simulink model "MSD_control"  (R2024b)
settings: Solver=ode4  StartTime=0.0  StopTime=10.0  FixedStep=1e-4  MaxStep=1e-3  RelTol=1e-3  EnableMultiTasking=on
values from neighbouring files (symbols this model uses):
  k_ref = 0.12    [MAIN_MSD_control.m]    (also in MAIN_slip_control.m)
  k_thresh = 0.001    [MAIN_MSD_control.m]    (also in MAIN_slip_control.m)
  Kd_high = 40    [MAIN_MSD_control.m]    (also in MAIN_slip_control.m = 5)
  Kd_low = 30    [MAIN_MSD_control.m]    (also in MAIN_slip_control.m = 5)
  Kd_thresh = 0/3.6    (= 0)    [MAIN_slip_control.m]
  Kp_high = 400    [MAIN_MSD_control.m]    (also in MAIN_slip_control.m = 500)
  Kp_low = 10    [MAIN_MSD_control.m]    (also in MAIN_slip_control.m = 100)
undefined symbols (not defined in the file or in its folder): Kp_thresh, par
libraries: simulink x3, Delft_Tyre_dtlib x1, Delft_Tyre_sm1glib x1
settings Model: Creator=bshyrokau  LastModifiedBy=nicvi
settings SolverCC: AlgebraicLoopSolver=TrustRegion
settings DataIOCC: SaveOutput=off  SignalLogging=off  DSMLogging=off  SaveTime=off  ReturnWorkspaceOutputs=off
settings OptimizationCC: ReuseModelBlockBuffer=off  LifeSpan=inf
settings DebuggingCC: UnconnectedInputMsg=warning  UnconnectedOutputMsg=warning  UnconnectedLineMsg=warning  AllowSymbolicDim=off  SFUnexpectedBacktrackingDiag=warning  SFNoUnconditionalDefaultTransitionDiag=warning  SFExecutionAtInitializationDiag=none  ArithmeticOperatorsInVariantConditions=warning
settings ModelReferenceCC: EnableRefExpFcnMdlSchedulingChecks=on  PropagateSignalLabelsOutOfModel=off
settings SFSimCC: SimUseLocalCustomCode=off  CustomCodeUndefinedFunction=UseInterfaceOnly
settings RTWCC: RTWUseLocalCustomCode=off  GPUComputeCapability=3.5  DLArmComputeVersion=19.05
settings CodeAppCC: StateflowObjectComments=on
settings GRTTargetCC: TargetLangStandard=C89/C90 (ANSI)
settings ConfigComp: CovMetricSettings=dw  CovSaveCumulativeToWorkspaceVar=on  CovSaveSingleToWorkspaceVar=on  CovExternalEMLEnable=off

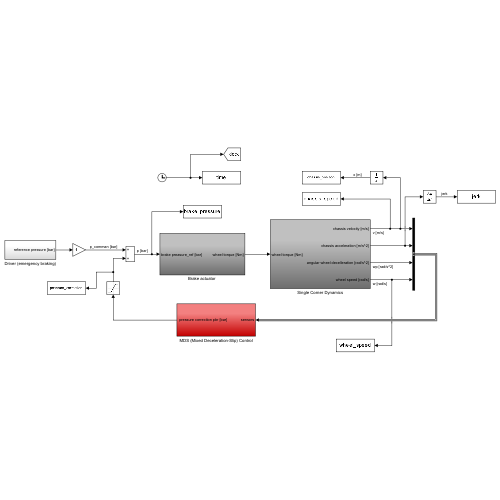
[thumbnail: Simulink's stored preview of the top-level diagram]
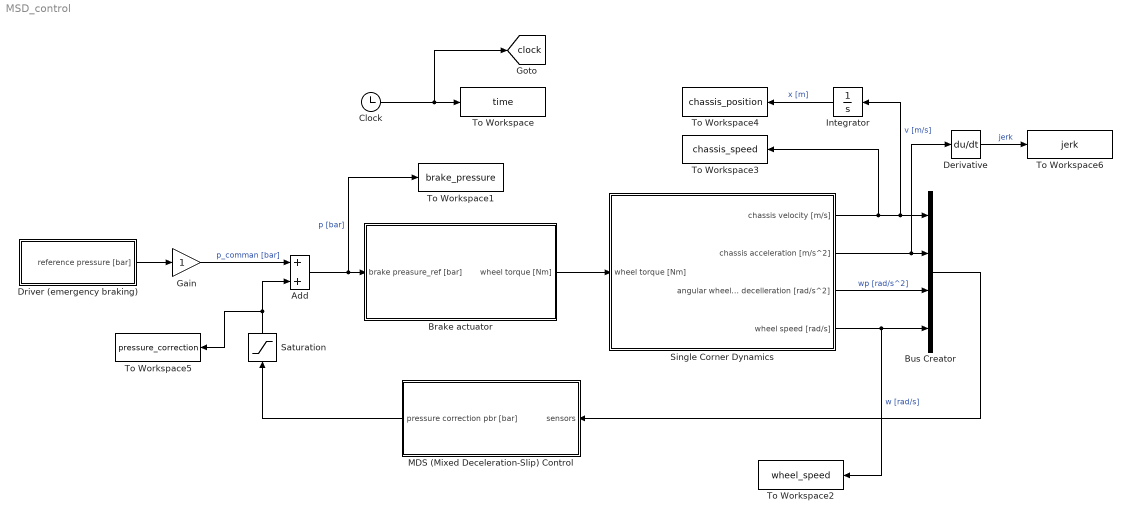
== system MSD_control ==
  Add : Sum
  "Brake actuator " : Subsystem
  Bus Creator : BusCreator  Inputs=4
  Clock : Clock
  Derivative : Derivative
  Driver (emergency braking) : Subsystem
  Gain : Gain
  Integrator : Integrator
  MDS (Mixed Deceleration-Slip) Control : Subsystem
  Saturation : Saturate  UpperLimit=0  LowerLimit=-100
  Single Corner Dynamics : Subsystem
  To Workspace : ToWorkspace  VariableName=time  SampleTime=-1
  To Workspace1 : ToWorkspace  VariableName=brake_pressure  SampleTime=-1
  To Workspace2 : ToWorkspace  VariableName=wheel_speed  SampleTime=-1
  To Workspace3 : ToWorkspace  VariableName=chassis_speed  SampleTime=-1
  To Workspace4 : ToWorkspace  VariableName=chassis_position  SampleTime=-1
  To Workspace5 : ToWorkspace  VariableName=pressure_correction  SampleTime=-1
  To Workspace6 : ToWorkspace  VariableName=jerk  SampleTime=-1
  tag scope: clock=global
  wires:
  "Brake actuator "/1(wheel torque [Nm]) -> Single Corner Dynamics/1(wheel torque [Nm])
  Add/1 -> To Workspace1/1, "Brake actuator "/1(brake preasure_ref [bar])  "p [bar]"
  MDS (Mixed Deceleration-Slip) Control/1(" pressure correction pbr [bar]") -> Saturation/1
  Single Corner Dynamics/1(chassis velocity [m/s]) -> Integrator/1, Bus Creator/1, To Workspace3/1  "v [m/s]"
  Single Corner Dynamics/3(angular wheel decelleration [rad/s^2]) -> Bus Creator/3  "wp [rad/s^2]"
  Single Corner Dynamics/4(wheel speed [rad/s]) -> Bus Creator/4, To Workspace2/1  "w [rad/s]"
  Bus Creator/1 -> MDS (Mixed Deceleration-Slip) Control/1(sensors)
  Driver (emergency braking)/1(reference pressure [bar]) -> Gain/1
  Gain/1 -> Add/1  "p_comman [bar]"
  Clock/1 -> [clock], To Workspace/1
  Saturation/1 -> To Workspace5/1, Add/2
  Integrator/1 -> To Workspace4/1  "x [m]"
  Single Corner Dynamics/2(chassis acceleration [m/s^2]) -> Derivative/1, Bus Creator/2
  Derivative/1 -> To Workspace6/1  "jerk"

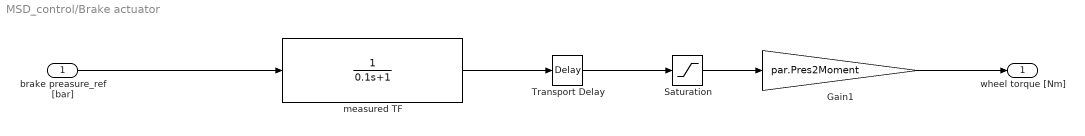
== system MSD_control/Brake actuator  ==
  brake preasure_ref [bar] : Inport
  " measured TF " : TransferFcn  Denominator=[0.1 1]
  Gain1 : Gain  Gain=par.Pres2Moment
  Saturation : Saturate  UpperLimit=par.max_pressure  LowerLimit=0
  Transport Delay : TransportDelay  DelayTime=0.06
  wheel torque [Nm] : Outport  VectorParamsAs1DForOutWhenUnconnected=off
  wires:
  Gain1/1 -> wheel torque [Nm]/1
  " measured TF "/1 -> Transport Delay/1
  Transport Delay/1 -> Saturation/1
  Saturation/1 -> Gain1/1
  brake preasure_ref [bar]/1 -> " measured TF "/1

== system MSD_control/Driver (emergency braking) ==
  Ramp : simulink/Sources/Ramp  slope=100  start=2  InitialOutput=0
  Saturation : Saturate  UpperLimit=100  LowerLimit=0
  reference pressure [bar] : Outport  VectorParamsAs1DForOutWhenUnconnected=off
  wires:
  Ramp/1 -> Saturation/1
  Saturation/1 -> reference pressure [bar]/1

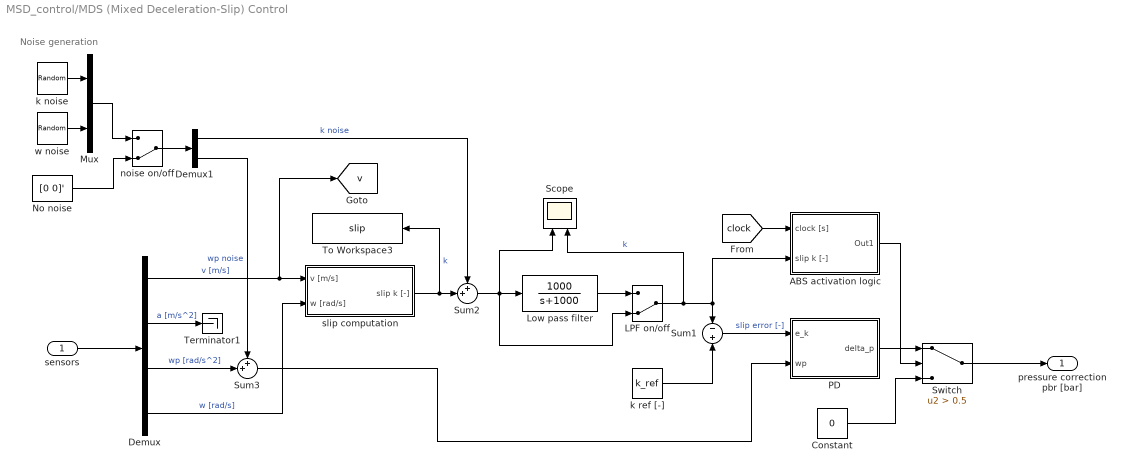
== system MSD_control/MDS (Mixed Deceleration-Slip) Control ==
  note: Noise generation
  sensors : Inport
  ABS activation logic : Subsystem
  Constant : Constant  Value=0
  Demux : Demux
  Demux1 : Demux  Outputs=2
  LPF on/off : ManualSwitch  CurrentSetting=0
  Low pass filter : TransferFcn  Numerator=[1000]  Denominator=[1 1000]
  Mux : Mux  Inputs=2
  No noise : Constant  Value=[0 0]'  OutDataTypeStr=Inherit: Inherit via back propagation
  PD : Subsystem
  Scope : Scope  NumInputPorts=2
  Sum1 : Sum  Inputs=-|+
  Sum2 : Sum  Inputs=++|
  Sum3 : Sum  Inputs=++|
  Switch : Switch  Criteria=u2 > Threshold  Threshold=0.5  SaturateOnIntegerOverflow=off  InputSameDT=off
  Terminator1 : Terminator
  To Workspace3 : ToWorkspace  VariableName=slip  SampleTime=-1
  k noise : UniformRandomNumber  Minimum=-0.025  Maximum=0.025  SampleTime=0
  k ref [-] : Constant  Value=k_ref
  noise on/off : ManualSwitch  CurrentSetting=0
  slip computation : Subsystem
  w noise : UniformRandomNumber  Minimum=-0.5  Maximum=0.5  SampleTime=0
  " pressure correction pbr [bar]" : Outport  VectorParamsAs1DForOutWhenUnconnected=off
  tag scope: v=global
  wires:
  sensors/1 -> Demux/1
  Demux/1 -> [v], slip computation/1(v [m/s])  "v [m/s]"
  Demux/2 -> Terminator1/1  "a [m/s^2]"
  Demux/4 -> slip computation/2(w [rad/s])  "w [rad/s]"
  Demux/3 -> Sum3/2  "wp [rad/s^2]"
  PD/1(delta_p) -> Switch/1
  k ref [-]/1 -> Sum1/2
  Sum1/1 -> PD/1(e_k)  "slip error [-]"
  Switch/1 -> " pressure correction pbr [bar]"/1
  ABS activation logic/1(Out1) -> Switch/2
  Constant/1 -> Switch/3
  [clock] -> ABS activation logic/1(clock [s])
  slip computation/1(slip k [-]) -> To Workspace3/1, Sum2/2  "k"
  w noise/1 -> Mux/2
  Mux/1 -> noise on/off/1
  k noise/1 -> Mux/1
  Demux1/2 -> Sum3/1  "wp noise"
  Demux1/1 -> Sum2/1  "k noise"
  noise on/off/1 -> Demux1/1
  No noise/1 -> noise on/off/2
  Sum3/1 -> PD/2(wp)
  Sum2/1 -> Scope/1, Low pass filter/1, LPF on/off/2
  Low pass filter/1 -> LPF on/off/1
  LPF on/off/1 -> Scope/2, ABS activation logic/2(slip k [-]), Sum1/1  "k"

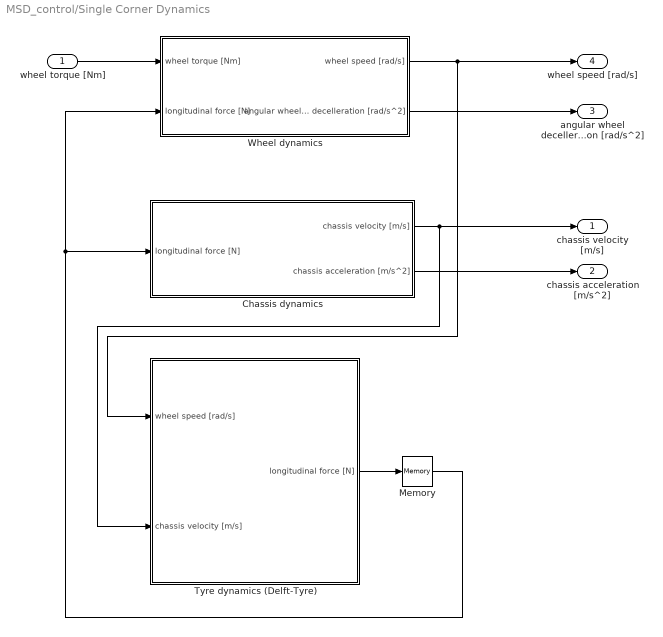
== system MSD_control/Single Corner Dynamics ==
  wheel torque [Nm] : Inport
  Chassis dynamics : Subsystem
  Memory : Memory
  Tyre dynamics (Delft-Tyre) : Subsystem
  Wheel dynamics : Subsystem
  chassis velocity [m/s] : Outport  VectorParamsAs1DForOutWhenUnconnected=off
  chassis acceleration [m/s^2] : Outport  Port=2  VectorParamsAs1DForOutWhenUnconnected=off
  angular wheel decelleration [rad/s^2] : Outport  Port=3  VectorParamsAs1DForOutWhenUnconnected=off
  wheel speed [rad/s] : Outport  Port=4  VectorParamsAs1DForOutWhenUnconnected=off
  wires:
  wheel torque [Nm]/1 -> Wheel dynamics/1(wheel torque [Nm])
  Wheel dynamics/1(wheel speed [rad/s]) -> Tyre dynamics (Delft-Tyre)/1(wheel speed [rad/s]), wheel speed [rad/s]/1
  Chassis dynamics/1(chassis velocity [m/s]) -> Tyre dynamics (Delft-Tyre)/2(chassis velocity [m/s]), chassis velocity [m/s]/1
  Tyre dynamics (Delft-Tyre)/1(longitudinal force [N]) -> Memory/1
  Memory/1 -> Wheel dynamics/2(longitudinal force [N]), Chassis dynamics/1(longitudinal force [N])
  Wheel dynamics/2(angular wheel decelleration [rad/s^2]) -> angular wheel decelleration [rad/s^2]/1
  Chassis dynamics/2(chassis acceleration [m/s^2]) -> chassis acceleration [m/s^2]/1

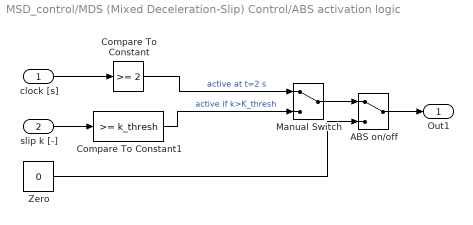
== system MSD_control/MDS (Mixed Deceleration-Slip) Control/ABS activation logic ==
  clock [s] : Inport
  slip k [-] : Inport  Port=2
  ABS on/off : ManualSwitch
  Compare To Constant : simulink/Logic and Bit Operations/Compare To Constant  relop=>=  const=2  OutDataTypeStr=boolean
  Compare To Constant1 : simulink/Logic and Bit Operations/Compare To Constant  relop=>=  const=k_thresh  OutDataTypeStr=boolean
  Manual Switch : ManualSwitch
  Zero : Constant  Value=0  OutDataTypeStr=Inherit: Inherit via back propagation
  Out1 : Outport
  wires:
  Compare To Constant1/1 -> Manual Switch/2  "active if k>K_thresh"
  Compare To Constant/1 -> Manual Switch/1  "active at t=2 s"
  slip k [-]/1 -> Compare To Constant1/1
  clock [s]/1 -> Compare To Constant/1
  Manual Switch/1 -> ABS on/off/1
  ABS on/off/1 -> Out1/1
  Zero/1 -> ABS on/off/2

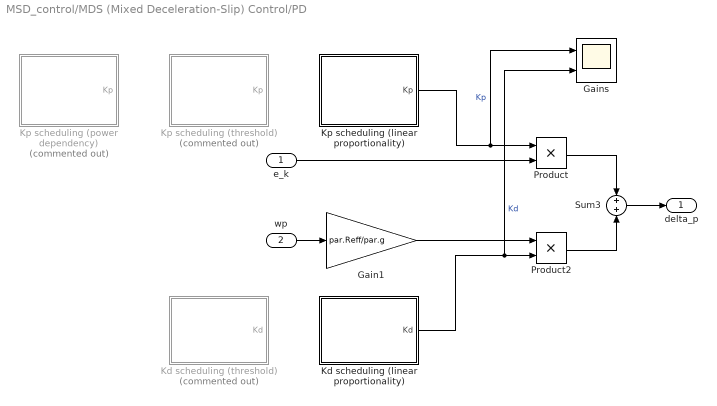
== system MSD_control/MDS (Mixed Deceleration-Slip) Control/PD ==
  e_k : Inport
  wp : Inport  Port=2
  Gain1 : Gain  Gain=par.Reff/par.g
  Gains : Scope  NumInputPorts=2
  Kd scheduling (linear proportionality) : Subsystem
  Kd scheduling (threshold) : Subsystem  Commented=on
  Kp scheduling (linear proportionality) : Subsystem
  Kp scheduling (power dependency) : Subsystem  Commented=on
  Kp scheduling (threshold) : Subsystem  Commented=on
  Product : Product
  Product2 : Product
  Sum3 : Sum  Inputs=+|+
  delta_p : Outport
  wires:
  Sum3/1 -> delta_p/1
  Product/1 -> Sum3/1
  e_k/1 -> Product/2
  wp/1 -> Gain1/1
  Gain1/1 -> Product2/1
  Kp scheduling (linear proportionality)/1(Kp) -> Gains/1, Product/1  "Kp"
  Kd scheduling (linear proportionality)/1(Kd) -> Product2/2, Gains/2  "Kd"
  Product2/1 -> Sum3/2

== system MSD_control/MDS (Mixed Deceleration-Slip) Control/slip computation ==
  v [m/s] : Inport
  w [rad/s] : Inport  Port=2
  Divide : Product  Inputs=*/
  Gain : Gain  Gain=par.Reff
  Sum : Sum  Inputs=-|+
  slip k [-] : Outport
  wires:
  v [m/s]/1 -> Sum/2, Divide/2
  Sum/1 -> Divide/1
  Divide/1 -> slip k [-]/1  "slip k [-]"
  w [rad/s]/1 -> Gain/1
  Gain/1 -> Sum/1  "v_wheel [m/s]"

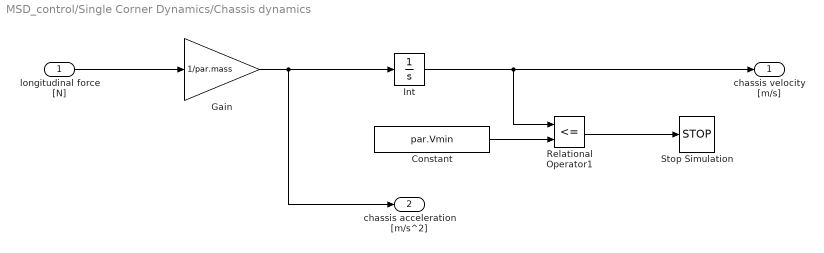
== system MSD_control/Single Corner Dynamics/Chassis dynamics ==
  longitudinal force [N] : Inport
  Constant : Constant  Value=par.Vmin
  Gain : Gain  Gain=1/par.mass
  Int : Integrator  InitialCondition=par.V0  LimitOutput=on  UpperSaturationLimit=200/3.6  LowerSaturationLimit=eps
  Relational Operator1 : RelationalOperator  Operator=<=
  Stop Simulation : Stop
  chassis velocity [m/s] : Outport  VectorParamsAs1DForOutWhenUnconnected=off
  chassis acceleration [m/s^2] : Outport  Port=2  VectorParamsAs1DForOutWhenUnconnected=off
  wires:
  longitudinal force [N]/1 -> Gain/1
  Int/1 -> Relational Operator1/1, chassis velocity [m/s]/1
  Gain/1 -> chassis acceleration [m/s^2]/1, Int/1
  Relational Operator1/1 -> Stop Simulation/1
  Constant/1 -> Relational Operator1/2

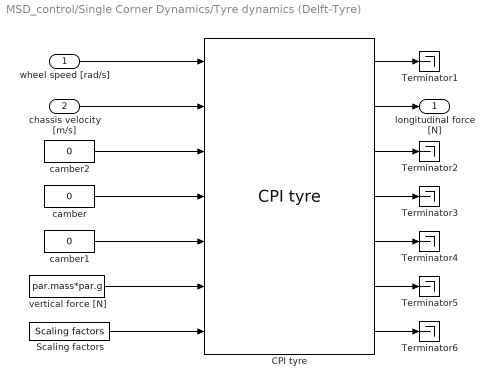
== system MSD_control/Single Corner Dynamics/Tyre dynamics (Delft-Tyre) ==
  wheel speed [rad/s] : Inport
  chassis velocity [m/s] : Inport  Port=2
  CPI tyre : Delft_Tyre_dtlib/Simulink/CPI tyre  Tag=CPI tyre  idtyre=1  tpfname='TNO_car205_60R15.tir'  side_mode=(3xxx) symmetric  dyn_mode=(xx1x) relaxation behaviour  mf_mode=(xxx1) longitudinal  use_mode=1e8  disp_debug=off
  Scaling factors : Delft_Tyre_sm1glib/SimMechanics 1G/Scaling factors  Tag=Scaling factors  LMUX=par.friction  LKX=1  LMUY=1  LKY=1  LKYC=1  LTR=1  LKZC=1
  Terminator{1..6} (6 alike) : Terminator
  camber : Constant  Value=0
  camber1 : Constant  Value=0
  camber2 : Constant  Value=0
  vertical force [N] : Constant  Value=par.mass*par.g
  longitudinal force [N] : Outport  VectorParamsAs1DForOutWhenUnconnected=off
  wires:
  Scaling factors/1 -> CPI tyre/7
  camber2/1 -> CPI tyre/3
  camber/1 -> CPI tyre/4
  CPI tyre/1 -> Terminator1/1
  CPI tyre/3 -> Terminator2/1
  CPI tyre/4 -> Terminator3/1
  CPI tyre/6 -> Terminator5/1
  CPI tyre/5 -> Terminator4/1
  camber1/1 -> CPI tyre/5
  chassis velocity [m/s]/1 -> CPI tyre/2
  wheel speed [rad/s]/1 -> CPI tyre/1
  CPI tyre/2 -> longitudinal force [N]/1
  vertical force [N]/1 -> CPI tyre/6
  CPI tyre/7 -> Terminator6/1

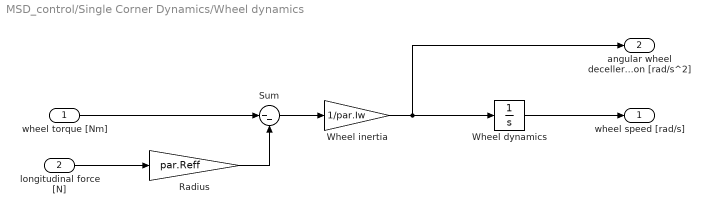
== system MSD_control/Single Corner Dynamics/Wheel dynamics ==
  wheel torque [Nm] : Inport
  longitudinal force [N] : Inport  Port=2
  Radius : Gain  Gain=par.Reff  SaturateOnIntegerOverflow=on  OutDataTypeStr=Inherit: Same as input  ParamDataTypeStr=Inherit: Same as input
  Sum : Sum  Inputs=|--  InputSameDT=on  SaturateOnIntegerOverflow=on  OutDataTypeStr=Inherit: Same as first input
  Wheel dynamics : Integrator  InitialCondition=par.V0/par.Reff  LimitOutput=on  UpperSaturationLimit=200/3.6/par.Reff  LowerSaturationLimit=eps
  Wheel inertia : Gain  Gain=1/par.Iw  SaturateOnIntegerOverflow=on  OutDataTypeStr=Inherit: Same as input  ParamDataTypeStr=Inherit: Same as input
  wheel speed [rad/s] : Outport  VectorParamsAs1DForOutWhenUnconnected=off
  angular wheel decelleration [rad/s^2] : Outport  Port=2  VectorParamsAs1DForOutWhenUnconnected=off
  wires:
  Wheel inertia/1 -> angular wheel decelleration [rad/s^2]/1, Wheel dynamics/1
  wheel torque [Nm]/1 -> Sum/1
  Wheel dynamics/1 -> wheel speed [rad/s]/1
  Sum/1 -> Wheel inertia/1
  longitudinal force [N]/1 -> Radius/1
  Radius/1 -> Sum/2

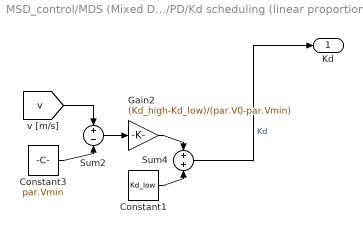
== system MSD_control/MDS (Mixed Deceleration-Slip) Control/PD/Kd scheduling (linear proportionality) ==
  Constant1 : Constant  Value=Kd_low
  Constant3 : Constant  Value=par.Vmin
  Gain2 : Gain  Gain=(Kd_high-Kd_low)/(par.V0-par.Vmin)
  Sum2 : Sum  Inputs=+|-
  Sum4 : Sum  Inputs=+|+
  Kd : Outport
  wires:
  [v] -> Sum2/1
  Gain2/1 -> Sum4/1
  Constant1/1 -> Sum4/2
  Constant3/1 -> Sum2/2
  Sum4/1 -> Kd/1  "Kd"
  Sum2/1 -> Gain2/1

== system MSD_control/MDS (Mixed Deceleration-Slip) Control/PD/Kd scheduling (threshold) ==
  Kd high v : Constant  Value=Kd_high
  Kd low v : Constant  Value=Kd_low  OutDataTypeStr=Inherit: Inherit via back propagation
  Switch2 : Switch  Criteria=u2 > Threshold  Threshold=Kd_thresh  SaturateOnIntegerOverflow=off  InputSameDT=off
  Kd : Outport
  wires:
  [v] -> Switch2/2
  Kd high v/1 -> Switch2/1
  Kd low v/1 -> Switch2/3
  Switch2/1 -> Kd/1  "Kd"

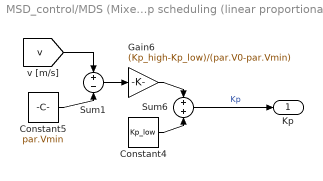
== system MSD_control/MDS (Mixed Deceleration-Slip) Control/PD/Kp scheduling (linear proportionality) ==
  Constant4 : Constant  Value=Kp_low
  Constant5 : Constant  Value=par.Vmin
  Gain6 : Gain  Gain=(Kp_high-Kp_low)/(par.V0-par.Vmin)
  Sum1 : Sum  Inputs=+|-
  Sum6 : Sum  Inputs=+|+
  Kp : Outport
  wires:
  Sum1/1 -> Gain6/1
  Gain6/1 -> Sum6/1
  [v] -> Sum1/1
  Constant5/1 -> Sum1/2
  Constant4/1 -> Sum6/2
  Sum6/1 -> Kp/1  "Kp"

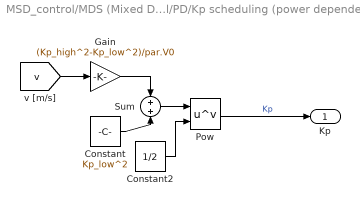
== system MSD_control/MDS (Mixed Deceleration-Slip) Control/PD/Kp scheduling (power dependency) ==
  Constant : Constant  Value=Kp_low^2
  Constant2 : Constant  Value=1/2
  Gain : Gain  Gain=(Kp_high^2-Kp_low^2)/par.V0
  Pow : Math  Operator=pow  RndMeth=Zero
  Sum : Sum  Inputs=+|+
  Kp : Outport
  wires:
  Pow/1 -> Kp/1  "Kp"
  Gain/1 -> Sum/1
  Constant2/1 -> Pow/2
  Sum/1 -> Pow/1
  Constant/1 -> Sum/2
  [v] -> Gain/1

== system MSD_control/MDS (Mixed Deceleration-Slip) Control/PD/Kp scheduling (threshold) ==
  Kp high v : Constant  Value=Kp_high
  Kp low v : Constant  Value=Kp_low
  Switch1 : Switch  Criteria=u2 > Threshold  Threshold=Kp_thresh  SaturateOnIntegerOverflow=off  InputSameDT=off
  Kp : Outport
  wires:
  Kp high v/1 -> Switch1/1
  Kp low v/1 -> Switch1/3
  [v] -> Switch1/2
  Switch1/1 -> Kp/1  "Kp"
